simulink model "Lab_2"  (R2021b)
settings: Solver=VariableStepAuto  StartTime=0.0  StopTime=10.0  RelTol=1e-3
libraries: spsRMSLib x4, spsPower3phInstantaneousLib x2, spsThreePhaseVIMeasurementLib x2, spsDistributedParametersLineLib x1, spsThreePhaseSeriesRLCLoadLib x1, spsThreePhaseSourceLib x1, spspowerguiLib x1
settings Model: Creator=coolk  LastModifiedBy=coolk

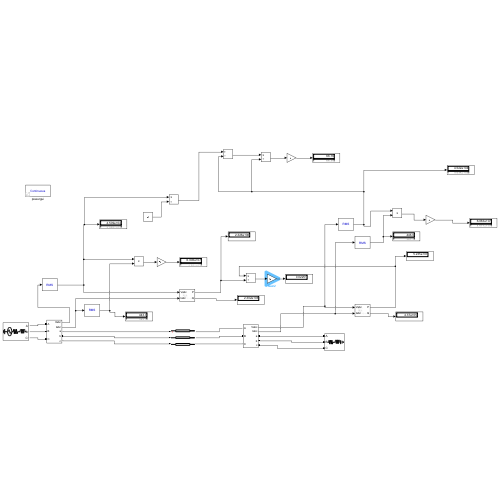
[thumbnail: Simulink's stored preview of the top-level diagram]
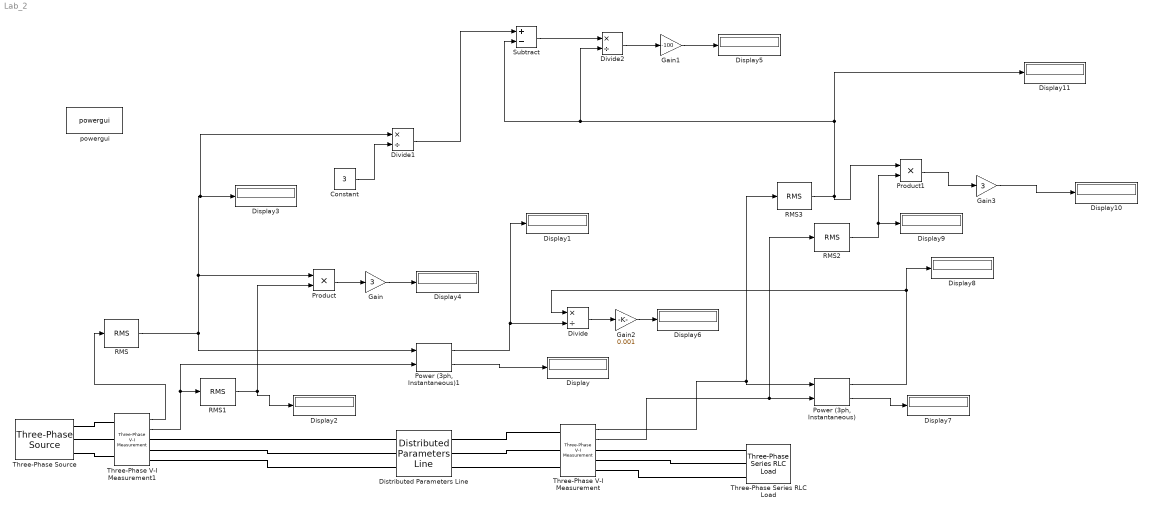
== system Lab_2 ==
  Constant : Constant  Value=3
  Display{,1..11} (12 alike) : Display
  Distributed Parameters Line : spsDistributedParametersLineLib/Distributed Parameters Line  Phases=3  Length=100  Frequency=50  Resistance=[0 0]  Inductance="[0.97e-3  0.99e-3]"  Capacitance=[11.5e-9 11.5e-9]  x1=[1.31169191280205e-11 75512.1617198579 75512.1617198579;314.159265358979 314.159265358979 314.159265358979;0.482000034660581 0.421051174655257 -1.14974515213964]  x2=[1.81898940354586e-11 72440.3503278715 72440.3503278716;314.159265358979 314.159265358979 314.159265358979;-0.106002568886986 0.124931708372476 -1.44586461842242]  x3=[8.31668949581372e-14 475.036921226407 475.036921226407;314.159265358979 314.159265358979 314.159265358979;2.6868190811189 -3.13429589399829 1.5780930863864]  x4=[2.1316282072803e-13 973.871422981789 973.87142298179;314.159265358979 314.159265358979 314.159265358979;-0.106002568886986 0.118732821309408 -1.45206350548549]  x5=0.00033741665637606  V1=[1.312e-11 7.551e+04 7.551e+04;314.2 314.2 314.2;0.482 0.4211 -1.15]  V2=[1.819e-11 7.244e+04 7.244e+04;314.2 314.2 314.2;-0.106 0.1249 -1.446]  I1=[8.317e-14 475 475;314.2 314.2 314.2;2.687 -3.134 1.578]  I2=[2.132e-13 973.9 973.9;314.2 314.2 314.2;-0.106 0.1187 -1.452]  nHarmo=1  Measurements=None  Decoupling=off  VsMag0=0  VrMag0=0  VsAngle0=0  VrAngle0=0  IsMag0=0  IrMag0=0  IsAngle0=0  IrAngle0=0
      settings: SourceProductBaseCode=PS
  Divide : Product  Inputs=*/
  Divide1 : Product  Inputs=*/
  Divide2 : Product  Inputs=*/
  Gain : Gain  Gain=3
  Gain1 : Gain  Gain=-100
  Gain2 : Gain  Gain=0.001
  Gain3 : Gain  Gain=3
  "Power (3ph, Instantaneous)" : spsPower3phInstantaneousLib/Power (3ph, Instantaneous)
  "Power (3ph, Instantaneous)1" : spsPower3phInstantaneousLib/Power (3ph, Instantaneous)
  Product : Product
  Product1 : Product
  RMS{,1..3} (4 alike) : spsRMSLib/RMS  TrueRMS=on  Freq=60  RMSInit=120  Ts=0
  Subtract : Sum  Inputs=+-
  Three-Phase Series RLC Load : spsThreePhaseSeriesRLCLoadLib/Three-Phase Series RLC Load  LConnTagsString=A|B|C  Configuration=Y (grounded)  NominalVoltage=1000  Vabc=[1e3 1e3 1e3]  Vabcp=[1e3 1e3 1e3]  NominalFrequency=60  UnbalancedPower=off  ActivePower=10e3  InductivePower=100  CapacitivePower=0  Pabc=[10e3 9e3 11e3]  QLabc=[100 90 110]  QCabc=[100 90 110]  Pabcp=[10e3 9e3 11e3]  QLabcp=[100 90 110]  QCabcp=[100 90 110]  Measurements=None  LoadType=constant Z
  Three-Phase V-I Measurement : spsThreePhaseVIMeasurementLib/Three-Phase V-I Measurement  VoltageMeasurement=phase-to-ground  SetLabelV=off  LabelV=Vabc  Vpu=off  VpuLL=off  CurrentMeasurement=yes  SetLabelI=off  LabelI=Iabc  Ipu=off  Pbase=100e6  Vbase=500e3  OutputType=Complex  PhasorSimulation=off  PSBequivalent=0
  Three-Phase V-I Measurement1 : spsThreePhaseVIMeasurementLib/Three-Phase V-I Measurement  VoltageMeasurement=phase-to-ground  SetLabelV=off  LabelV=Vabc  Vpu=off  VpuLL=off  CurrentMeasurement=yes  SetLabelI=off  LabelI=Iabc  Ipu=off  Pbase=100e6  Vbase=500e3  OutputType=Complex  PhasorSimulation=off  PSBequivalent=0
  Three-Phase Source : spsThreePhaseSourceLib/Three-Phase Source  InternalConnection=Yg  VoltagePhases=off  Voltage=76.21e3  PhaseAngle=0  Voltage_phases=[25e3 25e3 25e3]/sqrt(3)  PhaseAngles_phases=[0 -120 +120]  Frequency=50  NonIdealSource=on  SpecifyImpedance=off  Resistance=1  Inductance=4.444e-5  ShortCircuitLevel=100e6  BaseVoltage=25e3  XRratio=7  BusType=swing  Pref=10e3  Qref=0  Prefabc=[10e3, 10e3, 10e3]  Qrefabc=[0, 0, 0]  Qmin=-inf  Qmax=inf
  powergui : spspowerguiLib/powergui  Priority=1  SimulationMode=Continuous  SampleTime=50e-6  frequency=60  Iterations=50  frequencyindice=50  Pbase=100e6  ErrMax=1e-4  UnitsV=kV  UnitsW=MW  buscounter=0  FunctionMessages=off  echomessages=off  EnableUseOfTLC=off  CurrentSourceSwitches=off  DisableSnubberDevices=off  DisableRonSwitches=off  DisableVfSwitches=off  DisplayEquations=off  AutomaticDiscreteSolvers=off  SolverType=Tustin/Backward Euler (TBE)  Interpol=off  ExternalGateDelay=off  methode=off  Ts=100  x0status=blocks  SPID=on  SwTol=0  HookPort=off  NonlinearTolerance=1e-4  nMaxIteration=100  ContinueOnMaxIteration=off  RestoreLinks=warning  ResistiveCurrentMeasurement=off  Frange=[0:2:500]  Ylog=off  Xlog=on  ShowGrid=off  save=off  variable=ZData  structure=0  ZoomFFT=off  StartTime=0.0  cycles=1  DisplayStyle=1  fundamental=60  FreqAxis=off  MaxFrequency=1000  frequencyindicesteady=1  RmsSteady=1  display=off
  wires:
  Three-Phase V-I Measurement1/1 -> RMS/1
  Three-Phase V-I Measurement1/2 -> RMS1/1, "Power (3ph, Instantaneous)1"/2
  RMS/1 -> "Power (3ph, Instantaneous)1"/1, Product/1, Divide1/1, Display3/1
  "Power (3ph, Instantaneous)1"/2 -> Display/1
  RMS1/1 -> Display2/1, Product/2
  Constant/1 -> Divide1/2
  Divide1/1 -> Subtract/1
  Subtract/1 -> Divide2/1
  Product/1 -> Gain/1
  Gain/1 -> Display4/1
  Divide2/1 -> Gain1/1
  Gain1/1 -> Display5/1
  Divide/1 -> Gain2/1
  Gain2/1 -> Display6/1
  Three-Phase V-I Measurement/1 -> RMS3/1, "Power (3ph, Instantaneous)"/1
  Three-Phase V-I Measurement/2 -> RMS2/1, "Power (3ph, Instantaneous)"/2
  "Power (3ph, Instantaneous)"/2 -> Display7/1
  "Power (3ph, Instantaneous)"/1 -> Display8/1, Divide/1
  RMS2/1 -> Product1/2, Display9/1
  RMS3/1 -> Product1/1, Divide2/2, Subtract/2, Display11/1
  Gain3/1 -> Display10/1
  Product1/1 -> Gain3/1
  "Power (3ph, Instantaneous)1"/1 -> Display1/1, Divide/2
  connections:
  Three-Phase Source/RConn1 -- Three-Phase V-I Measurement1/LConn1
  Three-Phase Source/RConn2 -- Three-Phase V-I Measurement1/LConn2
  Three-Phase Source/RConn3 -- Three-Phase V-I Measurement1/LConn3
  Distributed Parameters Line/LConn1 -- Three-Phase V-I Measurement1/RConn1
  Distributed Parameters Line/LConn2 -- Three-Phase V-I Measurement1/RConn2
  Distributed Parameters Line/LConn3 -- Three-Phase V-I Measurement1/RConn3
  Three-Phase V-I Measurement/LConn1 -- Distributed Parameters Line/RConn1
  Three-Phase V-I Measurement/LConn2 -- Distributed Parameters Line/RConn2
  Three-Phase V-I Measurement/LConn3 -- Distributed Parameters Line/RConn3
  Three-Phase V-I Measurement/RConn1 -- Three-Phase Series RLC Load/LConn1
  Three-Phase V-I Measurement/RConn2 -- Three-Phase Series RLC Load/LConn2
  Three-Phase V-I Measurement/RConn3 -- Three-Phase Series RLC Load/LConn3
